simulink model "ACE_II_AC_DCMotor"  (R2025b)
settings: Solver=ode15s  StartTime=0.0  StopTime=50  FixedStep=0.01  MaxStep=0.2  RelTol=1e-3
undefined symbols (not defined in the file): b, J, Km, La, q0, q1, Ra, T
libraries: simulink x1
settings Model: Creator=Felix  LastModifiedBy=Felix

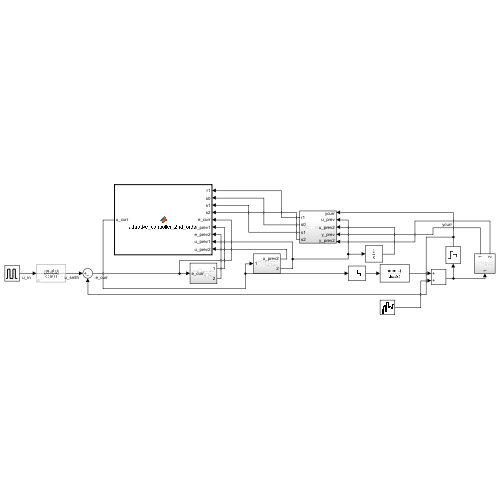
[thumbnail: Simulink's stored preview of the top-level diagram]
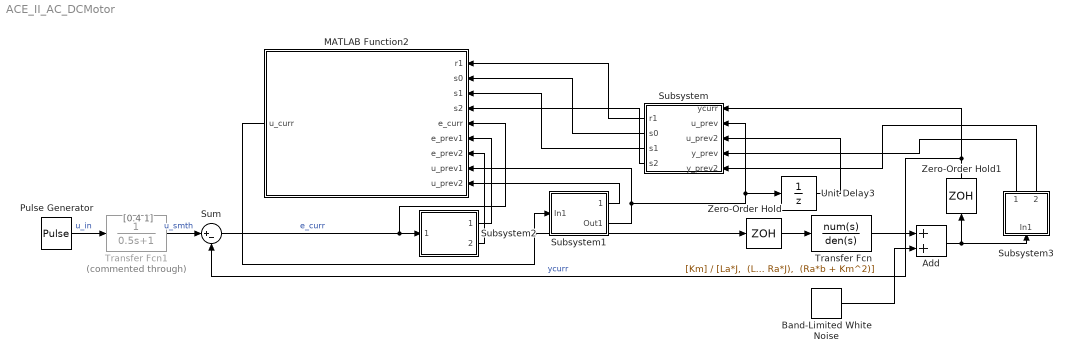
== system ACE_II_AC_DCMotor ==
  note: [0.4 1]
  Add : Sum
  Band-Limited White Noise : simulink/Sources/Band-Limited White Noise  Cov=[0.001]  Ts=T  seed=[23341]
  MATLAB Function2 : MATLAB Function  TreatAsAtomicUnit=on
  Pulse Generator : DiscretePulseGenerator  PulseType=Time based  Amplitude=10  Period=20  PulseWidth=50
  Subsystem : Subsystem
  Subsystem1 : Subsystem
  Subsystem2 : Subsystem
  Subsystem3 : Subsystem
  Sum : Sum  Inputs=|+-
  Transfer Fcn : TransferFcn  Numerator=[Km]  Denominator="[La*J,  (La*b + Ra*J),  (Ra*b + Km^2)]"
  Transfer Fcn1 : TransferFcn  Commented=through  Denominator=[0.5 1]
  Unit Delay3 : UnitDelay  SampleTime=-1  HasFrameUpgradeWarning=on
  Zero-Order Hold : ZeroOrderHold  SampleTime=-1
  Zero-Order Hold1 : ZeroOrderHold  SampleTime=-1
  wires:
  Zero-Order Hold/1 -> Transfer Fcn/1
  Transfer Fcn/1 -> Add/1
  Band-Limited White Noise/1 -> Add/2
  Add/1 -> Zero-Order Hold1/1, Subsystem3/1(In1)
  MATLAB Function2/1(u_curr) -> Subsystem1/1(In1), Zero-Order Hold/1
  Zero-Order Hold1/1 -> Subsystem/1(ycurr), Sum/2  "ycurr"
  Sum/1 -> Subsystem2/1(e_curr), MATLAB Function2/5(e_curr)  "e_curr"
  Unit Delay3/1 -> Subsystem/3(u_prev2)
  Subsystem/1(r1) -> MATLAB Function2/1(r1)
  Subsystem/2(s0) -> MATLAB Function2/2(s0)
  Subsystem/3(s1) -> MATLAB Function2/3(s1)
  Subsystem/4(s2) -> MATLAB Function2/4(s2)
  Subsystem1/2(Out1) -> MATLAB Function2/8(u_prev1), Subsystem/2(u_prev), Unit Delay3/1
  Subsystem1/1(u_prev2) -> MATLAB Function2/9(u_prev2)
  Subsystem2/1(Out1) -> MATLAB Function2/6(e_prev1)
  Subsystem2/2(Out2) -> MATLAB Function2/7(e_prev2)
  Subsystem3/1(Out1) -> Subsystem/4(y_prev)
  Subsystem3/2(Out2) -> Subsystem/5(y_prev2)
  Pulse Generator/1 -> Transfer Fcn1/1  "u_in"
  Transfer Fcn1/1 -> Sum/1  "u_smth"

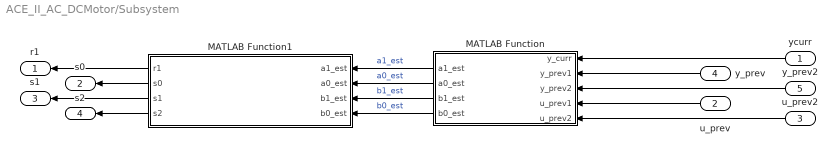
== system ACE_II_AC_DCMotor/Subsystem ==
  ycurr : Inport
  u_prev : Inport  Port=2
  u_prev2 : Inport  Port=3
  y_prev : Inport  Port=4
  y_prev2 : Inport  Port=5
  MATLAB Function : MATLAB Function  TreatAsAtomicUnit=on
  MATLAB Function1 : MATLAB Function  TreatAsAtomicUnit=on
  r1 : Outport
  s0 : Outport  Port=2
  s1 : Outport  Port=3
  s2 : Outport  Port=4
  wires:
  MATLAB Function/4(b0_est) -> MATLAB Function1/4(b0_est)  "b0_est"
  y_prev/1 -> MATLAB Function/2(y_prev1)
  MATLAB Function/2(a0_est) -> MATLAB Function1/2(a0_est)  "a0_est"
  ycurr/1 -> MATLAB Function/1(y_curr)
  u_prev/1 -> MATLAB Function/4(u_prev1)
  MATLAB Function/1(a1_est) -> MATLAB Function1/1(a1_est)  "a1_est"
  MATLAB Function/3(b1_est) -> MATLAB Function1/3(b1_est)  "b1_est"
  MATLAB Function1/1(r1) -> r1/1
  MATLAB Function1/2(s0) -> s0/1
  MATLAB Function1/4(s2) -> s2/1
  MATLAB Function1/3(s1) -> s1/1
  u_prev2/1 -> MATLAB Function/5(u_prev2)
  y_prev2/1 -> MATLAB Function/3(y_prev2)

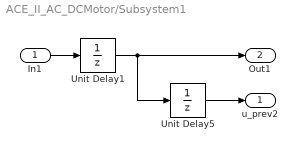
== system ACE_II_AC_DCMotor/Subsystem1 ==
  In1 : Inport
  Unit Delay1 : UnitDelay  SampleTime=-1  HasFrameUpgradeWarning=on
  Unit Delay5 : UnitDelay  SampleTime=-1  HasFrameUpgradeWarning=on
  u_prev2 : Outport
  Out1 : Outport  Port=2
  wires:
  In1/1 -> Unit Delay1/1
  Unit Delay5/1 -> u_prev2/1
  Unit Delay1/1 -> Out1/1, Unit Delay5/1

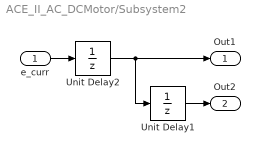
== system ACE_II_AC_DCMotor/Subsystem2 ==
  e_curr : Inport
  Unit Delay1 : UnitDelay  SampleTime=-1  HasFrameUpgradeWarning=on
  Unit Delay2 : UnitDelay  SampleTime=-1  HasFrameUpgradeWarning=on
  Out1 : Outport
  Out2 : Outport  Port=2
  wires:
  Unit Delay2/1 -> Out1/1, Unit Delay1/1
  e_curr/1 -> Unit Delay2/1
  Unit Delay1/1 -> Out2/1

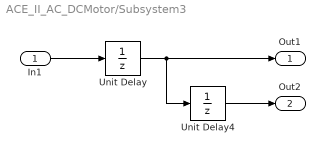
== system ACE_II_AC_DCMotor/Subsystem3 ==
  In1 : Inport
  Unit Delay : UnitDelay  SampleTime=-1  HasFrameUpgradeWarning=on
  Unit Delay4 : UnitDelay  SampleTime=-1  HasFrameUpgradeWarning=on
  Out1 : Outport
  Out2 : Outport  Port=2
  wires:
  Unit Delay/1 -> Unit Delay4/1, Out1/1
  Unit Delay4/1 -> Out2/1
  In1/1 -> Unit Delay/1

== matlab function ACE_II_AC_DCMotor/Subsystem/MATLAB Function1 ==
  data: a1_est input; a0_est input; b1_est input; b0_est input; q0 parameter; q1 parameter; r1 output; s0 output; s1 output; s2 output
function [r1, s0, s1, s2] = pole_placement_controller(a1_est, a0_est, b1_est, b0_est, q0, q1)
    
    % 1. PERSISTENT MEMORY FOR SAFETY
    % If the matrix becomes unsolvable during startup, we use the last known good values.
    persistent r1_prev s0_prev s1_prev s2_prev initialized
    if isempty(initialized)
        r1_prev = 0; s0_prev = 0; s1_prev = 0; s2_prev = 0;
        initialized = true;
    end

    % 2. BUILD THE SYLVESTER MATRIX (M)
    M = [ 1,               b1_est, 0,      0;
          a1_est - 1,      b0_est, b1_est, 0;
          a0_est - a1_est, 0,      b0_est, b1_est;
         -a0_est,          0,      0,      b0_est ];
         
    % 3. BUILD THE TARGET VECTOR (Y)
    % We place your two desired poles (q1, q0) and place the remaining 
    % two observer poles at the origin (0) to keep the response fast.
    Y = [ q1 + 1 - a1_est;
          q0 + a1_est - a0_est;
          a0_est;
          0 ];
          
    % 4. SOLVE THE MATRIX
    % We check the determinant to ensure the matrix isn't singular 
    % (which can happen during the first few noisy milliseconds of simulation)
    if abs(det(M)) > 1e-4
        X = M \ Y; % Matrix left division solves M*X = Y
        
        r1 = X(1);
        s0 = X(2);
        s1 = X(3);
        s2 = X(4);
        
        % Save for next loop
        r1_prev = r1; s0_prev = s0; s1_prev = s1; s2_prev = s2;
    else
        % If math fails, use the safe previous values
        r1 = r1_prev; s0 = s0_prev; s1 = s1_prev; s2 = s2_prev;
    end
end

== matlab function ACE_II_AC_DCMotor/Subsystem/MATLAB Function ==
  data: a1_est output; y_curr input; y_prev1 input; a0_est output; b1_est output; y_prev2 input; b0_est output; u_prev1 input; u_prev2 input
function [a1_est, a0_est, b1_est, b0_est] = rls_estimator(y_curr, y_prev1, y_prev2, u_prev1, u_prev2)
    persistent P xe initialized
    
    if isempty(initialized)
        P = 100 * eye(4);           % Now a 4x4 matrix for 4 parameters
        xe = [-1.5; 0.5; 0.1; 0.1]; % Initial guess for [a1; a0; b1; b0]
        initialized = true;
    end
    
    alpha = 1.0; % Forgetting factor
    
    % 3. RECURSIVE LEAST SQUARES MATH
    % The measurement vector now looks at t-1 AND t-2
    C = [-y_prev1, -y_prev2, u_prev1, u_prev2];
    
    % Calculate the Kalman Gain (L)
    % Because C is 1x4 and P is 4x4, the denominator is still a scalar!
    denominator = (C * P * C') + alpha;
    L = (P * C') / denominator;
    
    % Calculate the error between actual motor speed and prediction
    y_prediction = C * xe;
    error = y_curr - y_prediction;
    
    % Update the 4 parameter estimates based on the error
    xe = xe + L * error;
    
    % Update the 4x4 Covariance matrix for the next step
    P = (eye(4) - L * C) * P / alpha;
    
    % 4. ASSIGN OUTPUTS
    a1_est = xe(1);
    a0_est = xe(2);
    b1_est = xe(3);
    b0_est = xe(4);
end

== matlab function ACE_II_AC_DCMotor/MATLAB Function2 ==
  data: r1 input; s0 input; s1 input; s2 input; u_curr output; e_curr input; e_prev1 input; e_prev2 input; u_prev1 input; u_prev2 input
function u_curr = adaptive_controller_2nd_order(r1, s0, s1, s2, e_curr, e_prev1, e_prev2, u_prev1, u_prev2)

    % 1. The 2nd-Order Control Law
    % u(k) = (1 - r1)*u(k-1) + r1*u(k-2) + s0*e(k) + s1*e(k-1) + s2*e(k-2)
    u_curr = (1 - r1) * u_prev1 + r1 * u_prev2 + (s0 * e_curr) + (s1 * e_prev1) + (s2 * e_prev2);

    % 2. Hardware Saturation (Clamp to +/- 12 Volts)
    % This is still mandatory to protect your simulated (and physical) driver
    % max_volts = 12;
    % if u_calc > max_volts
    %     u_curr = max_volts;
    % elseif u_calc < -max_volts
    %     u_curr = -max_volts;
    % else
    %     u_curr = u_calc;
    % end
end
